simulink model "model_idealacc_2018b"  (R2018b)
settings: Solver=FixedStepAuto  StartTime=0.0  StopTime=10000  FixedStep=1  RelTol=1e-3
values from neighbouring files (symbols this model uses):
  r_start = [aux_p(1:3) r_0 aux_p(4:end)]    [Five_chasers_init.m]
  v_start = [aux_v(1:3) v_0 aux_v(4:end)]    [Five_chasers_init.m]
settings Model: Creator=Benny Rievers  LastModifiedBy=Riya Bhattacharjee
settings SFSimCC: SimUseLocalCustomCode=off
settings RTWCC: RTWUseLocalCustomCode=off

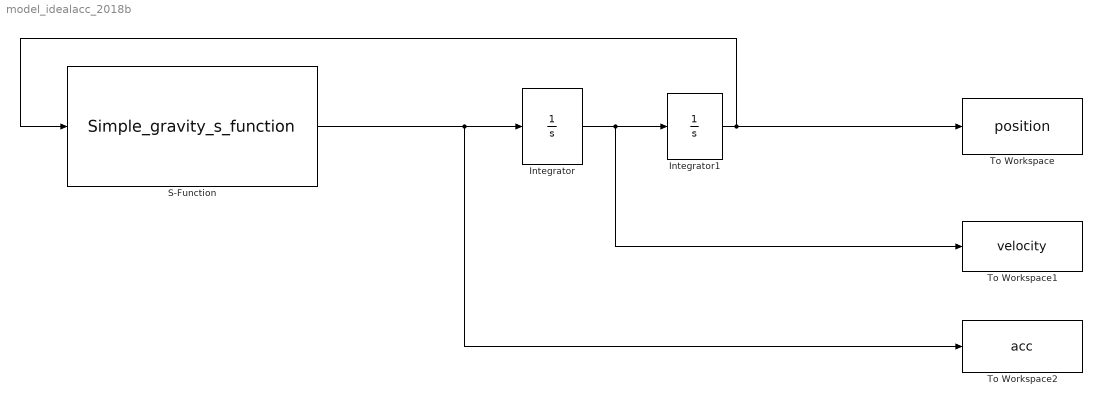
== system model_idealacc_2018b ==
  Integrator : Integrator  InitialCondition=v_start
  Integrator1 : Integrator  InitialCondition=r_start
  S-Function : S-Function  FunctionName=Simple_gravity_s_function  SFunctionDeploymentMode=off  EnableBusSupport=off
  To Workspace : ToWorkspace  VariableName=position  SampleTime=-1
  To Workspace1 : ToWorkspace  VariableName=velocity  SampleTime=-1
  To Workspace2 : ToWorkspace  VariableName=acc  SampleTime=-1
  wires:
  Integrator/1 -> To Workspace1/1, Integrator1/1
  S-Function/1 -> To Workspace2/1, Integrator/1
  Integrator1/1 -> S-Function/1, To Workspace/1
